simulink model "ad_maskparam"  (R2015b)
settings: Solver=FixedStepDiscrete  SolverMode=SingleTasking  StartTime=0.0  StopTime=10.0  RelTol=1e-3
PreLoadFcn:
  | H=[1 0 3 0 1]/4
  | pipeline=0
libraries: simulink x1
settings Model: Creator=at-mt  LastModifiedBy=amatsumo
settings DataIOCC: SaveFormat=Array  SignalLoggingSaveFormat=ModelDataLogs  SaveOutput=off  SignalLogging=off  SaveTime=off
settings OptimizationCC: BlockReduction=off  ConditionallyExecuteInputs=off  DefaultParameterBehavior=Inlined  ExpressionDepthLimit=2147483647
settings DebuggingCC: AlgebraicLoopMsg=error  UnderspecifiedInitializationDetection=Classic  MergeDetectMultiDrivingBlocksExec=none  SolverPrmCheckMsg=warning  SingleTaskRateTransMsg=error  FcnCallInpInsideContextMsg=UseLocalSettings  StateNameClashWarn=warning
settings HardwareCC: ProdBitPerPointer=32  ProdLargestAtomicFloat=None  ProdIntDivRoundTo=Undefined  ProdEndianess=Unspecified  ProdWordSize=32  ProdHWDeviceType=ASIC/FPGA->ASIC/FPGA  ProdEqTarget=off
settings GRTTargetCC: GeneratePreprocessorConditionals=Disable all  CombineOutputUpdateFcns=off  GRTInterface=on
settings ConfigComp: CovModelRefEnable=Off  CovSFcnEnable=off

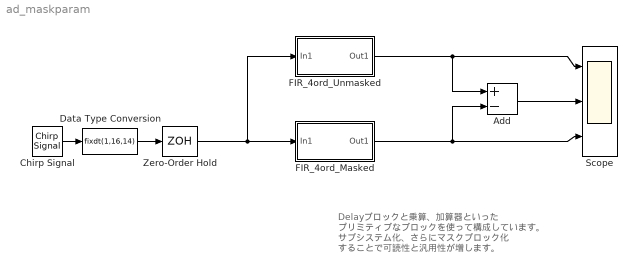
== system ad_maskparam ==
  note: Delayブロックと乗算、加算器といった
      | プリミティブなブロックを使って構成しています。
      | サブシステム化、さらにマスクブロック化
      | することで可読性と汎用性が増します。
  Add : Sum  Inputs=+-
  Chirp Signal : simulink/Sources/Chirp Signal  f1=10  T=10  f2=500
  Data Type Conversion : DataTypeConversion  OutDataTypeStr=fixdt(1,16,14)  RndMeth=Nearest
  FIR_4ord_Masked : Subsystem  mask(4次FIRフィルタ){H=[1 0 3 0 1]/4, pipeline=0}
      mask prompts: H "Coefficients(5個)"; pipeline "Pipeline Level"
      mask help: フィルタの係数（5個）と積和演算後のパイプラインレベル（FF数）を設定して下さい。
      mask init:
      | str1 = ['H = ', num2str(H)];
      | str2 = ['Pipeline Level = ', num2str(pipeline)];
      | strvcat(str1,str2)
      mask Help: FIRフィルタのヘルプドキュメントを記述します。
  FIR_4ord_Unmasked : Subsystem
  Scope : Scope  NumInputPorts=3
  Zero-Order Hold : ZeroOrderHold  SampleTime=1/1000
  wires:
  Chirp Signal/1 -> Data Type Conversion/1
  Zero-Order Hold/1 -> FIR_4ord_Unmasked/1(In1), FIR_4ord_Masked/1(In1)
  Add/1 -> Scope/2
  Data Type Conversion/1 -> Zero-Order Hold/1
  FIR_4ord_Unmasked/1(Out1) -> Add/1, Scope/1
  FIR_4ord_Masked/1(Out1) -> Add/2, Scope/3

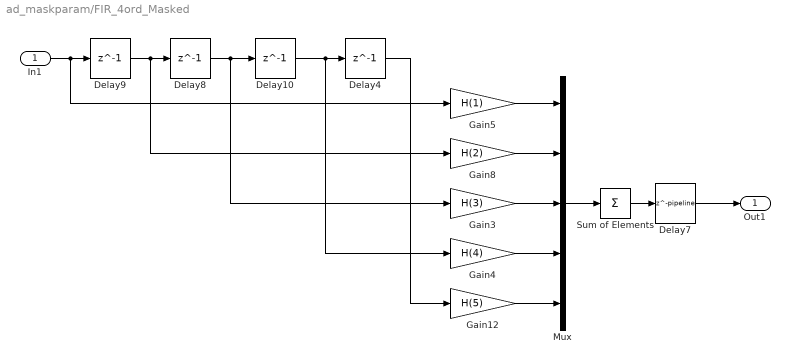
== system ad_maskparam/FIR_4ord_Masked ==
  In1 : Inport
  Delay{4,8..10} (4 alike) : Delay  DelayLength=1  InitialCondition=0  InputProcessing=Inherited
  Delay7 : Delay  DelayLength=pipeline  InitialCondition=0  InputProcessing=Inherited
  Gain12 : Gain  Gain=H(5)  RndMeth=Nearest  OutDataTypeStr=Inherit: Same as input
  Gain3 : Gain  Gain=H(3)  RndMeth=Nearest  OutDataTypeStr=Inherit: Same as input
  Gain4 : Gain  Gain=H(4)  RndMeth=Nearest  OutDataTypeStr=Inherit: Same as input
  Gain5 : Gain  Gain=H(1)  RndMeth=Nearest  OutDataTypeStr=Inherit: Same as input
  Gain8 : Gain  Gain=H(2)  RndMeth=Nearest  OutDataTypeStr=Inherit: Same as input
  Mux : Mux  Inputs=5
  Sum of Elements : Sum  Inputs=+  RndMeth=Nearest
  Out1 : Outport
  wires:
  Sum of Elements/1 -> Delay7/1
  Gain12/1 -> Mux/5
  Gain4/1 -> Mux/4
  Gain3/1 -> Mux/3
  Gain8/1 -> Mux/2
  Gain5/1 -> Mux/1
  Delay4/1 -> Gain12/1
  Mux/1 -> Sum of Elements/1
  Delay8/1 -> Delay10/1, Gain3/1
  Delay9/1 -> Delay8/1, Gain8/1
  Delay10/1 -> Delay4/1, Gain4/1
  In1/1 -> Gain5/1, Delay9/1
  Delay7/1 -> Out1/1

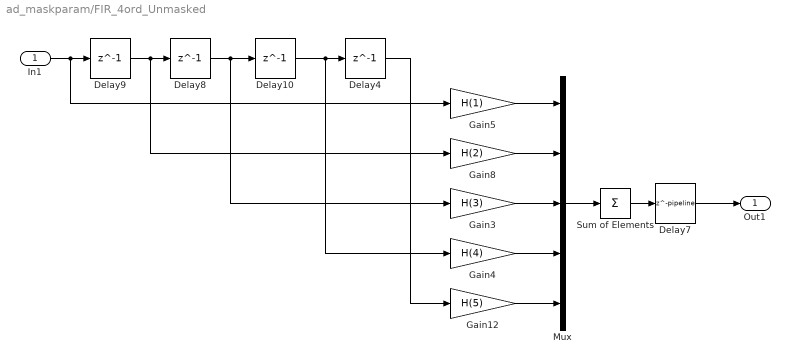
== system ad_maskparam/FIR_4ord_Unmasked ==
  In1 : Inport
  Delay{4,8..10} (4 alike) : Delay  DelayLength=1  InitialCondition=0  InputProcessing=Inherited
  Delay7 : Delay  DelayLength=pipeline  InitialCondition=0  InputProcessing=Inherited
  Gain12 : Gain  Gain=H(5)  RndMeth=Nearest  OutDataTypeStr=Inherit: Same as input
  Gain3 : Gain  Gain=H(3)  RndMeth=Nearest  OutDataTypeStr=Inherit: Same as input
  Gain4 : Gain  Gain=H(4)  RndMeth=Nearest  OutDataTypeStr=Inherit: Same as input
  Gain5 : Gain  Gain=H(1)  RndMeth=Nearest  OutDataTypeStr=Inherit: Same as input
  Gain8 : Gain  Gain=H(2)  RndMeth=Nearest  OutDataTypeStr=Inherit: Same as input
  Mux : Mux  Inputs=5
  Sum of Elements : Sum  Inputs=+  RndMeth=Nearest
  Out1 : Outport
  wires:
  Delay7/1 -> Out1/1
  In1/1 -> Delay9/1, Gain5/1
  Delay10/1 -> Gain4/1, Delay4/1
  Delay9/1 -> Gain8/1, Delay8/1
  Delay8/1 -> Gain3/1, Delay10/1
  Mux/1 -> Sum of Elements/1
  Delay4/1 -> Gain12/1
  Gain5/1 -> Mux/1
  Gain8/1 -> Mux/2
  Gain3/1 -> Mux/3
  Gain4/1 -> Mux/4
  Gain12/1 -> Mux/5
  Sum of Elements/1 -> Delay7/1
